simulink model "groundContact"  (R2026a)
settings: configuration reference "standardSILConfiguraitonParams" (kept outside this file)
undefined symbols (not defined in the file or in its folder): stepSize_s
libraries: matrix_library x3
settings Model: Creator=GTAR  LastModifiedBy=Edison Altamirano
settings ConfigSetRef: SourceName=standardSILConfiguraitonParams  SourceLocation=Base Workspace

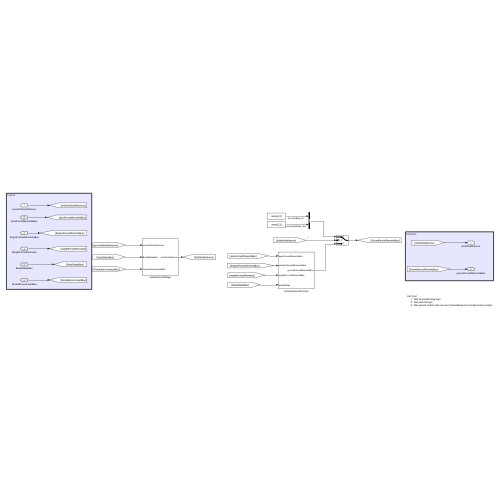
[thumbnail: Simulink's stored preview of the top-level diagram]
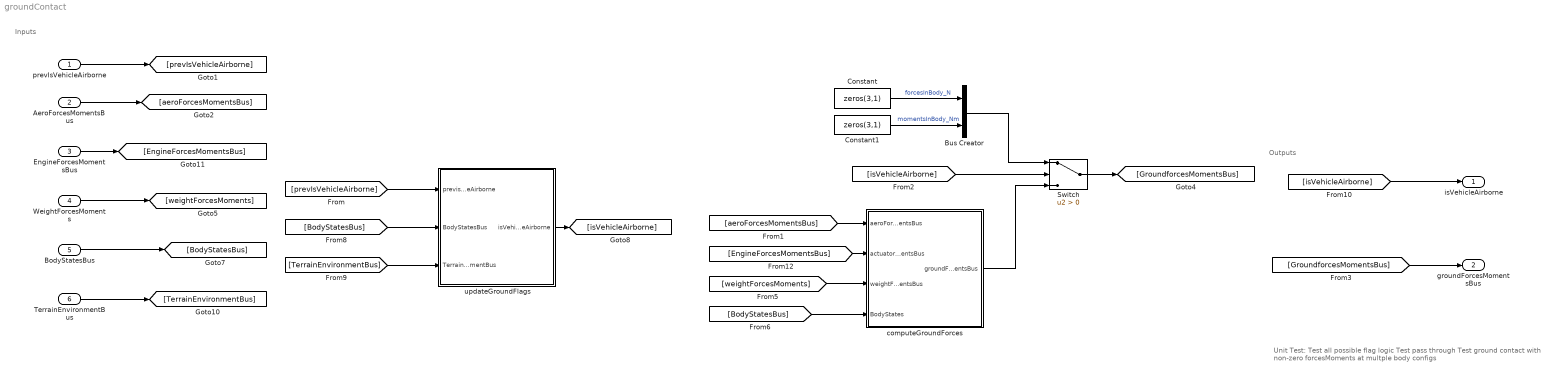
== system groundContact ==
  note: Unit Test:
      | Test all possible flag logic
      | Test pass through
      | Test ground contact with non-zero forcesMoments at multple body configs
  note: Outputs
  note: Inputs
  prevIsVehicleAirborne : Inport  OutDataTypeStr=boolean
  AeroForcesMomentsBus : Inport  Port=2  OutDataTypeStr=Bus: ComponentForcesMomentsBus
  EngineForcesMomentsBus : Inport  Port=3  OutDataTypeStr=Bus: ComponentForcesMomentsBus
  WeightForcesMoments : Inport  Port=4  OutDataTypeStr=Bus: ComponentForcesMomentsBus
  BodyStatesBus : Inport  Port=5  OutDataTypeStr=Bus: BodyStateBus
  TerrainEnvironmentBus : Inport  Port=6  OutDataTypeStr=Bus: TerrainEnvironmentBus
  Bus Creator : BusCreator  Inputs=2  OutDataTypeStr=Bus: ComponentForcesMomentsBus
  Constant : Constant  Value=zeros(3,1)
  Constant1 : Constant  Value=zeros(3,1)
  Switch : Switch  Criteria=u2 > Threshold  SaturateOnIntegerOverflow=off  InputSameDT=off
  computeGroundForces : Subsystem
  updateGroundFlags : Subsystem
  isVehicleAirborne : Outport  OutDataTypeStr=boolean
  groundForcesMomentsBus : Outport  Port=2  OutDataTypeStr=Bus: ComponentForcesMomentsBus
  wires:
  AeroForcesMomentsBus/1 -> [aeroForcesMomentsBus]
  prevIsVehicleAirborne/1 -> [prevIsVehicleAirborne]
  [prevIsVehicleAirborne] -> updateGroundFlags/1(previsVehicleAirborne)
  [isVehicleAirborne] -> Switch/2
  WeightForcesMoments/1 -> [weightForcesMoments]
  BodyStatesBus/1 -> [BodyStatesBus]
  [GroundforcesMomentsBus] -> groundForcesMomentsBus/1
  [BodyStatesBus] -> updateGroundFlags/2(BodyStatesBus)
  [TerrainEnvironmentBus] -> updateGroundFlags/3(TerrainEnvironmentBus)
  updateGroundFlags/1(isVehicleAirborne) -> [isVehicleAirborne]
  [isVehicleAirborne] -> isVehicleAirborne/1
  TerrainEnvironmentBus/1 -> [TerrainEnvironmentBus]
  EngineForcesMomentsBus/1 -> [EngineForcesMomentsBus]
  [aeroForcesMomentsBus] -> computeGroundForces/1(aeroForcesMomentsBus)
  [EngineForcesMomentsBus] -> computeGroundForces/2(actuatorForcesMomentsBus)
  [weightForcesMoments] -> computeGroundForces/3(weightForcesMomentsBus)
  [BodyStatesBus] -> computeGroundForces/4(BodyStates)
  Constant/1 -> Bus Creator/1  "forcesInBody_N"
  Constant1/1 -> Bus Creator/2  "momentsInBody_Nm"
  computeGroundForces/1(groundForcesMomentsBus) -> Switch/3
  Switch/1 -> [GroundforcesMomentsBus]
  Bus Creator/1 -> Switch/1

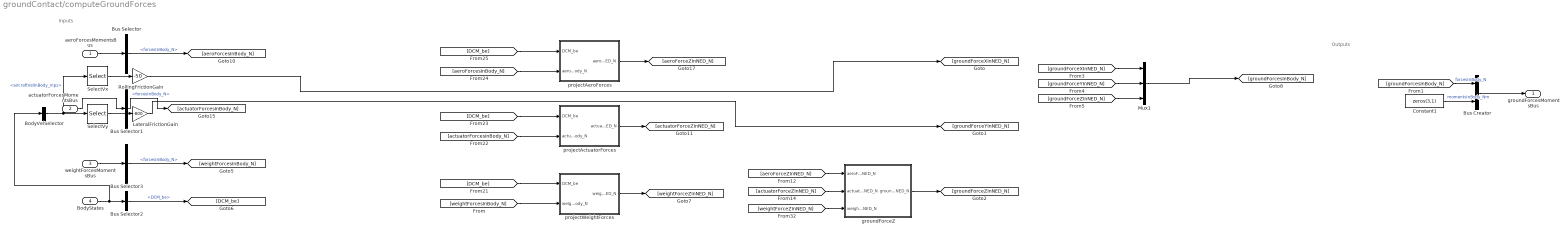
== system groundContact/computeGroundForces ==
  note: Inputs
  note: Outputs
  aeroForcesMomentsBus : Inport  OutDataTypeStr=Bus: ComponentForcesMomentsBus
  actuatorForcesMomentsBus : Inport  Port=2  OutDataTypeStr=Bus: ComponentForcesMomentsBus
  weightForcesMomentsBus : Inport  Port=3  OutDataTypeStr=Bus: ComponentForcesMomentsBus
  BodyStates : Inport  Port=4  OutDataTypeStr=Bus: BodyStateBus
  BodyVelSelector : BusSelector  OutputSignals=aircraftVelInBody_mps
  Bus Creator : BusCreator  Inputs=2  OutDataTypeStr=Bus: ComponentForcesMomentsBus
  Bus Selector : BusSelector  OutputSignals=forcesInBody_N
  Bus Selector1 : BusSelector  OutputSignals=forcesInBody_N
  Bus Selector2 : BusSelector  OutputSignals=DCM_be
  Bus Selector3 : BusSelector  OutputSignals=forcesInBody_N
  Constant1 : Constant  Value=zeros(3,1)
  LateralFrictionGain : Gain  Gain=-800
  Mux1 : Mux  Inputs=3
  RollingFrictionGain : Gain  Gain=-50
  SelectVx : Selector  IndexOptions=Index vector (dialog)  Indices=[1]  OutputSizes=1
  SelectVy : Selector  IndexOptions=Index vector (dialog)  Indices=[2]  OutputSizes=1
  groundForceZ : Subsystem
  projectActuatorForces : Subsystem
  projectAeroForces : Subsystem
  projectWeightForces : Subsystem
  groundForcesMomentsBus : Outport  OutDataTypeStr=Bus: ComponentForcesMomentsBus
  wires:
  aeroForcesMomentsBus/1 -> Bus Selector/1
  groundForceZ/1(groundForceZInNED_N) -> [groundForceZInNED_N]
  [aeroForceZInNED_N] -> groundForceZ/1(aeroForceZInNED_N)
  [actuatorForceZInNED_N] -> groundForceZ/2(actuatorForceZInNED_N)
  [groundForceXInNED_N] -> Mux1/1
  [groundForceYInNED_N] -> Mux1/2
  [groundForceZInNED_N] -> Mux1/3
  actuatorForcesMomentsBus/1 -> Bus Selector1/1
  Bus Selector/1 -> [aeroForcesInBody_N]  "<forcesInBody_N>"
  BodyStates/1 -> BodyVelSelector/1, Bus Selector2/1
  Bus Selector2/1 -> [DCM_be]  "<DCM_be>"
  [groundForcesInBody_N] -> Bus Creator/1  "forcesInBody_N"
  weightForcesMomentsBus/1 -> Bus Selector3/1
  Bus Selector3/1 -> [weightForcesInBody_N]  "<forcesInBody_N>"
  [DCM_be] -> projectWeightForces/1(DCM_be)
  [weightForcesInBody_N] -> projectWeightForces/2(weightForcesInBody_N)
  projectWeightForces/1(weightForceZInNED_N) -> [weightForceZInNED_N]
  projectActuatorForces/1(actuatorForceZInNED_N) -> [actuatorForceZInNED_N]
  [actuatorForcesInBody_N] -> projectActuatorForces/2(actuatorForcesInBody_N)
  [DCM_be] -> projectActuatorForces/1(DCM_be)
  [DCM_be] -> projectAeroForces/1(DCM_be)
  [aeroForcesInBody_N] -> projectAeroForces/2(aeroForcesInBody_N)
  projectAeroForces/1(aeroForceZInNED_N) -> [aeroForceZInNED_N]
  Bus Selector1/1 -> [actuatorForcesInBody_N]  "<forcesInBody_N>"
  [weightForceZInNED_N] -> groundForceZ/3(weightForceZInNED_N)
  Bus Creator/1 -> groundForcesMomentsBus/1
  Constant1/1 -> Bus Creator/2  "momentsInBody_Nm"
  BodyVelSelector/1 -> SelectVy/1, SelectVx/1  "<aircraftVelInBody_mps>"
  SelectVx/1 -> RollingFrictionGain/1
  SelectVy/1 -> LateralFrictionGain/1
  RollingFrictionGain/1 -> [groundForceXInNED_N]
  LateralFrictionGain/1 -> [groundForceYInNED_N]
  Mux1/1 -> [groundForcesInBody_N]

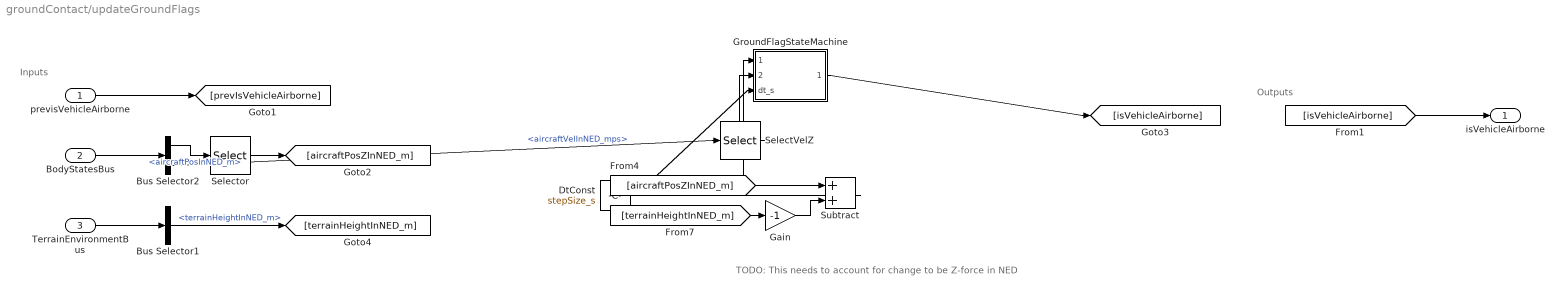
== system groundContact/updateGroundFlags ==
  note: TODO: This needs to account for change to be Z-force in NED
  note: Outputs
  note: Inputs
  previsVehicleAirborne : Inport  OutDataTypeStr=boolean
  BodyStatesBus : Inport  Port=2  OutDataTypeStr=Bus: BodyStateBus
  TerrainEnvironmentBus : Inport  Port=3  OutDataTypeStr=Bus: TerrainEnvironmentBus
  Bus Selector1 : BusSelector  OutputSignals=terrainHeightInNED_m
  Bus Selector2 : BusSelector  OutputSignals=aircraftPosInNED_m,aircraftVelInNED_mps
  DtConst : Constant  Value=stepSize_s
  Gain : Gain  Gain=-1
  GroundFlagStateMachine : MATLAB Function  TreatAsAtomicUnit=on
  SelectVelZ : Selector  InputPortWidth=3  IndexOptions=Index vector (dialog)  Indices=[3]  OutputSizes=1
  Selector : Selector  InputPortWidth=3  IndexOptions=Index vector (dialog)  Indices=3  OutputSizes=1
  Subtract : Sum
  isVehicleAirborne : Outport  OutDataTypeStr=boolean
  wires:
  TerrainEnvironmentBus/1 -> Bus Selector1/1
  previsVehicleAirborne/1 -> [prevIsVehicleAirborne]
  BodyStatesBus/1 -> Bus Selector2/1
  Selector/1 -> [aircraftPosZInNED_m]
  [isVehicleAirborne] -> isVehicleAirborne/1
  Bus Selector1/1 -> [terrainHeightInNED_m]  "<terrainHeightInNED_m>"
  [aircraftPosZInNED_m] -> Subtract/1
  [terrainHeightInNED_m] -> Gain/1
  Subtract/1 -> GroundFlagStateMachine/1(heightDiff_m)
  Gain/1 -> Subtract/2
  Bus Selector2/1 -> Selector/1  "<aircraftPosInNED_m>"
  Bus Selector2/2 -> SelectVelZ/1  "<aircraftVelInNED_mps>"
  SelectVelZ/1 -> GroundFlagStateMachine/2(velZ_mps)
  DtConst/1 -> GroundFlagStateMachine/3(dt_s)
  GroundFlagStateMachine/1(isAirborne) -> [isVehicleAirborne]

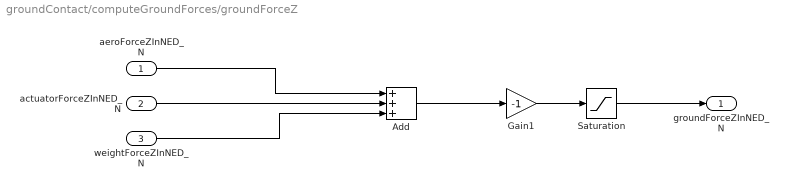
== system groundContact/computeGroundForces/groundForceZ ==
  aeroForceZInNED_N : Inport
  actuatorForceZInNED_N : Inport  Port=2
  weightForceZInNED_N : Inport  Port=3
  Add : Sum  Inputs=+++
  Gain1 : Gain  Gain=-1
  Saturation : Saturate  UpperLimit=0  LowerLimit=-inf
  groundForceZInNED_N : Outport
  wires:
  Add/1 -> Gain1/1
  aeroForceZInNED_N/1 -> Add/1
  actuatorForceZInNED_N/1 -> Add/2
  Gain1/1 -> Saturation/1
  weightForceZInNED_N/1 -> Add/3
  Saturation/1 -> groundForceZInNED_N/1

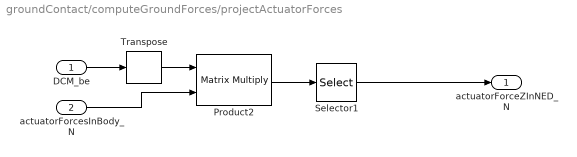
== system groundContact/computeGroundForces/projectActuatorForces ==
  DCM_be : Inport
  actuatorForcesInBody_N : Inport  Port=2
  Product2 : Product  Multiplication=Matrix(*)
  Selector1 : Selector  InputPortWidth=3  IndexOptions=Index vector (dialog)  Indices=[3]  OutputSizes=1
  Transpose : matrix_library/Transpose
  actuatorForceZInNED_N : Outport
  wires:
  actuatorForcesInBody_N/1 -> Product2/2
  Product2/1 -> Selector1/1
  Selector1/1 -> actuatorForceZInNED_N/1
  DCM_be/1 -> Transpose/1
  Transpose/1 -> Product2/1

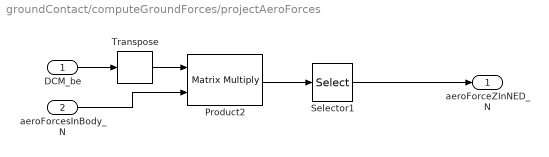
== system groundContact/computeGroundForces/projectAeroForces ==
  DCM_be : Inport
  aeroForcesInBody_N : Inport  Port=2
  Product2 : Product  Multiplication=Matrix(*)
  Selector1 : Selector  InputPortWidth=3  IndexOptions=Index vector (dialog)  Indices=[3]  OutputSizes=1
  Transpose : matrix_library/Transpose
  aeroForceZInNED_N : Outport
  wires:
  Transpose/1 -> Product2/1
  DCM_be/1 -> Transpose/1
  Selector1/1 -> aeroForceZInNED_N/1
  Product2/1 -> Selector1/1
  aeroForcesInBody_N/1 -> Product2/2

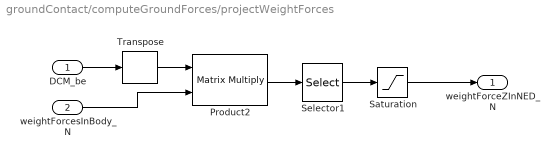
== system groundContact/computeGroundForces/projectWeightForces ==
  DCM_be : Inport
  weightForcesInBody_N : Inport  Port=2
  Product2 : Product  Multiplication=Matrix(*)
  Saturation : Saturate  UpperLimit=Inf  LowerLimit=0
  Selector1 : Selector  InputPortWidth=3  IndexOptions=Index vector (dialog)  Indices=[3]  OutputSizes=1
  Transpose : matrix_library/Transpose
  weightForceZInNED_N : Outport
  wires:
  Transpose/1 -> Product2/1
  DCM_be/1 -> Transpose/1
  Saturation/1 -> weightForceZInNED_N/1
  Product2/1 -> Selector1/1
  Selector1/1 -> Saturation/1
  weightForcesInBody_N/1 -> Product2/2

== matlab function groundContact/updateGroundFlags/GroundFlagStateMachine ==
  data: heightDiff_m input; isAirborne output; velZ_mps input; dt_s input
function isAirborne = GroundFlagStateMachine(heightDiff_m, velZ_mps, dt_s)
%#codegen
persistent airborneState climbTimer_s landTimer_s
if isempty(airborneState)
    airborneState = false;
    climbTimer_s = 0;
    landTimer_s = 0;
end

climbHeightThresh_m = -0.05;   % NED, negative = above terrain
climbVelThresh_mps  = -0.10;   % NED, negative = climbing
climbSustain_s      = 0.5;     % must hold for this long before latching airborne
landHeightThresh_m  = -0.02;   % must be back within this of terrain
landSustain_s       = 0.3;     % must hold for this long before resetting to grounded

if ~airborneState
    if heightDiff_m < climbHeightThresh_m && velZ_mps < climbVelThresh_mps
        climbTimer_s = climbTimer_s + dt_s;
    else
        climbTimer_s = 0;
    end
    if climbTimer_s >= climbSustain_s
        airborneState = true;
        landTimer_s = 0;
    end
else
    if heightDiff_m > landHeightThresh_m
        landTimer_s = landTimer_s + dt_s;
    else
        landTimer_s = 0;
    end
    if landTimer_s >= landSustain_s
        airborneState = false;
        climbTimer_s = 0;
    end
end

isAirborne = airborneState;
end
